simulink model "closed_loop_control_system_model"  (R2015a)
settings: Solver=ode45  StartTime=0.0  StopTime=1  RelTol=1e-3
values from neighbouring files (symbols this model uses):
  i_ep = op.States(3).x    [linearize_model.m]
  Kd = lqrd(A,B,Q,R,Ts)    [linearize_model.m]
  u_ep = op.Inputs(1).u    [linearize_model.m]
  z_ep = op.States(1).x    [linearize_model.m]
settings Model: Creator=Student  LastModifiedBy=Student
settings DataIOCC: LimitDataPoints=off

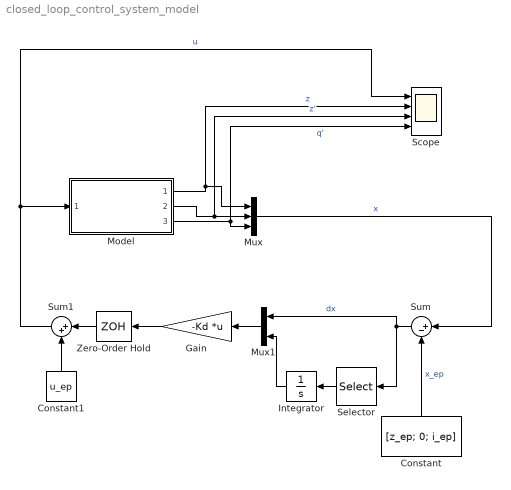
== system closed_loop_control_system_model ==
  Constant : Constant  Value=[z_ep; 0; i_ep]
  Constant1 : Constant  Value=u_ep
  Gain : Gain  Gain=-Kd  Multiplication=Matrix(K*u) (u vector)
  Integrator : Integrator
  Model : ModelReference  ModelNameDialog=plant_model_for_linearization  SimulationMode=Normal  ModelReferenceVersion=1.10  CopyOfModelName=plant_model_for_linearization  DefaultDataLogging=on
  Mux : Mux  Inputs=3
  Mux1 : Mux  Inputs=2
  Scope : Scope  NumInputPorts=4
      settings: ShowLegends=on  YMin=-5~-5~-5~-5  YMax=5~5~5~5  SaveName=ModelData
  Selector : Selector  InputPortWidth=3  Indices=[1]
  Sum : Sum  Inputs=|+-
  Sum1 : Sum  Inputs=|++
  Zero-Order Hold : ZeroOrderHold  SampleTime=0.001
  wires:
  Sum1/1 -> Model/1, Scope/1  "u"
  Model/1 -> Scope/2, Mux/1  "z"
  Model/2 -> Mux/2, Scope/3  "z'"
  Model/3 -> Mux/3, Scope/4  "q'"
  Mux/1 -> Sum/1  "x"
  Constant/1 -> Sum/2  "x_ep"
  Sum/1 -> Mux1/1, Selector/1  "dx"
  Gain/1 -> Zero-Order Hold/1
  Constant1/1 -> Sum1/2
  Zero-Order Hold/1 -> Sum1/1
  Selector/1 -> Integrator/1
  Mux1/1 -> Gain/1
  Integrator/1 -> Mux1/2
